simulink model "CreateMPC_FirstPrinciples"  (R2016a)
settings: Solver=VariableStepAuto  StartTime=0.0  StopTime=3000  RelTol=1e-3
values from neighbouring files (symbols this model uses):
  A = [a11 a12 a13 a14; a21 a22 a23 a24; a31 a32 a33 a34; a41 a42 a43 a44]    [LoadModel_FirstPrinciples.m]
  B = [b11 b12; b21 b22; b31 b32; b41 b42]    [LoadModel_FirstPrinciples.m]
  C = [0 0 1 0; 0 0 0 1]    [LoadModel_FirstPrinciples.m]
  D = [0 0; 0 0]    [LoadModel_FirstPrinciples.m]
libraries: mpclib x1
settings Model: Creator=tiago  LastModifiedBy=tiago

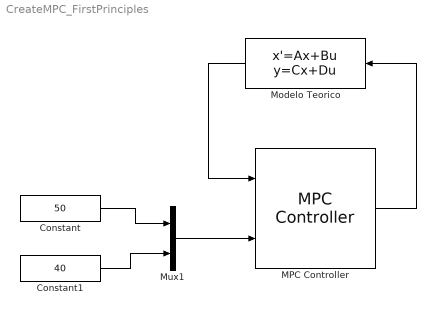
== system CreateMPC_FirstPrinciples ==
  Constant : Constant  Value=50
  Constant1 : Constant  Value=40
  MPC Controller : mpclib/MPC Controller  SCDEnableBlockLinearizationSpecification=on  mpcobj=mpc1  is_multiple=0  enable_value=0  return_u0=off  ref_from_ws=off  ref_signal_name=[]  ref_preview=off  md_from_ws=off  md_signal_name=[]  md_preview=off  from_project=off  project_file=MPCtask.mat  md_inport=off  mv_inport=off  cost_outport=off  return_sequence=off  return_qpstatus=off  return_state=off  state_inport=off  lims_inport=off  ywt_inport=off  is_designfromscratch=0  uwt_inport=off  duwt_inport=off  rhoeps_inport=off  uref_inport=off  n_ts=7  n_mv=2  n_md=1  n_ud=0  n_mo=2  n_uo=0  BlockDataType=double  SampleTimeInherited=off  switch_inport=off
  Modelo Teorico : StateSpace  A=A  B=B  C=C  D=D  X0=0
  Mux1 : Mux  Inputs=2
  wires:
  Constant/1 -> Mux1/1
  Constant1/1 -> Mux1/2
  Mux1/1 -> MPC Controller/2
  MPC Controller/1 -> Modelo Teorico/1
  Modelo Teorico/1 -> MPC Controller/1
